simulink model "meat_1024pt_bee2"  (Simulink 6.2)
settings: Solver=ode45  StartTime=0.0  StopTime=60000  RelTol=1e-3
undefined symbols (not defined in the file): BEE2_usr, bit_rev, pfb_coeff_gen_calc
libraries: xbsIndex_r3 x1083, casper_library x93, xps_library x28
(part 1 of 8)
settings Model: LastModifiedBy=siemion
settings DebuggingCC: SolverPrmCheckMsg=warning

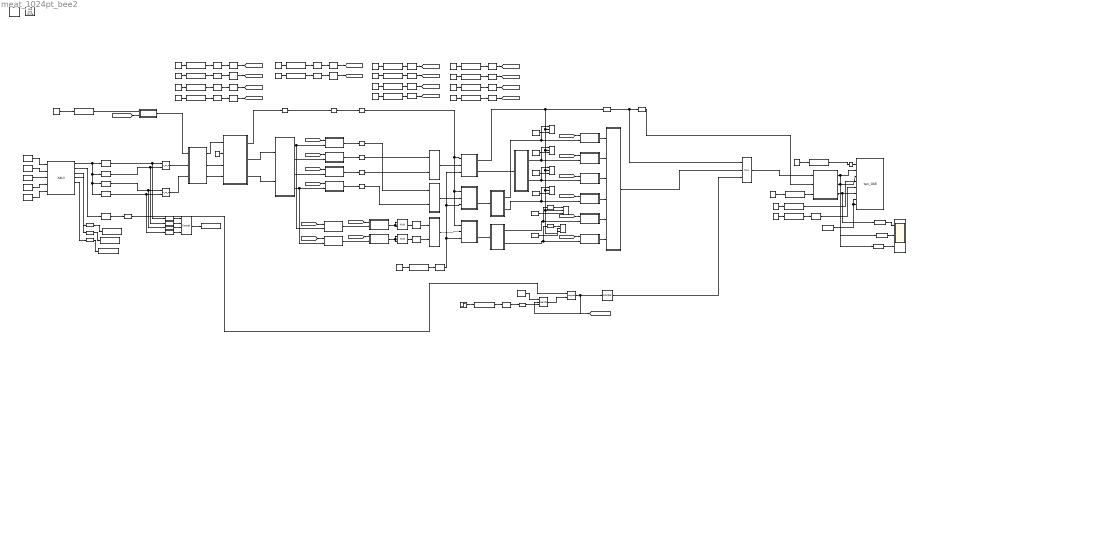
== system meat_1024pt_bee2 ==
  note: left
  note: ATA Kurtosis Machine
      | Author: Andrew Siemion
      | Author: Peter McMahon
      | Version: 1.0
      | August 2009
  note: n * LCM(taps*clksperFFT=4*1024=2048,
      | clksperacc=(acclen+1)*veclen=5*2048=10240)=20480
  note: XAUI Output:
      |
      | outofband[0]: 100PPS
      | outofband[1]: 1PPS
      |
      | data[0-7]: Pol 1 I
      | data[8-15]: Pol 1 Q
      | data[16-23]: Pol 2 I
      | data[24-31]: Pol 2 Q
      | data[31-63]: unused
  note: min acclen for serializer = # of parallel inputs
  note: XAUI Scope
      | Outputs raw bits from XAUI so you can measure voltage levels
  note: ARM/PPS Reset Circuit
      | 1. User sets ARM high at half-second
      | 2. 1PPS arrives.
      | 3. PPSARMReset signal goes high for one clock on the 1PPS
      | 4. ARM is reset, and won't go high again until user brings it low then high
  note: Unsigned, 18-bits, b.p. at 12
      | Coefficient by which to scale the output of the Stokes Detector.
  note: Extract 8 bits from 32
      | (latency: 1)
      | Don't delay valid since we will prepend a counter
      | and extend valid for one clock
  note: When "valid" goes high, it's the start of a
      | packet, so insert a counter.
      |
      | Note that since the bitselect_i subsystems each have a delay of 1,
      | valid goes high 1 clock before the data arrives.
  note: Need valid to be high while data is valid (1024 clocks), and
      | one extra clock for the "header" (counter). Total clocks: 1025.
  note: end-of-frame goes high for the last clock
      | that valid is high. This is a requirement for
      | the 10GbE block to work.
  note: ** Sending out data every second clock.
      | 10GbE tx_data input is 64 bits wide.
      | We only produce 32-bits of data per clock.
      | Therefore we must buffer 32-bits every second clock
      | and concat it with the current data output to get 64-bits
      | every second clock. The tx_valid line is modified to
      | accommodate this.
  note: Intended usage:
      | Connect to 108MHz bandwidth beamformer.
      | Input: I,Q 108MSa/sec, dual polarization.
      |   i.e. 8-bits I, 8-bits Q, x2 pol = 32 bits
      | Runs synchronously (i.e. assumes 32-bits
      | arrives from XAUI every FPGA clock)
  note: Selects which 8-bits from 32 are outputted.
      | 0 is lowest 8-bits.
      | 3 is highest 8-bits.
  note: Powers are unsigned and cross-terms are signed.
      | Hence we have to use separate accumulators for
      | them.
  note: Unsigned, 18-bits, b.p. at 12
      | Coefficient by which to scale the output of the Stokes Detector.
  note: Packet Size is in bytes / eight
  " System Generator" : xbsIndex_r3/ System Generator  Tag=genX  xilinxfamily=Virtex2P  part=xc2vp50  speed=-7  package=ff1152  synthesis_tool=XST  directory=./meat_1024pt_lwip_reg/sysgen  testbench=off  simulink_period=1  sysclk_period=8  incr_netlist=off  trim_vbits=Everywhere in SubSystem  dbl_ovrd=According to Block Masks  core_generation=According to Block Masks  run_coregen=off  deprecated_control=off  eval_field=0
      settings: AttributesFormatString=System\nGenerator
  Constant : Constant  Value=4000
  Constant1 : Constant  Value=4000
  Constant{10,15..17} (4 alike) : Constant  Value=0
  Constant{3..6,11..12} (6 alike) : Constant  Value=2^12
  Constant2 : Constant  Value=2
  Constant7 : Constant
  Constant8 : Constant
  Constant9 : Constant
  Convert : xbsIndex_r3/Convert  arith_type=Unsigned  n_bits=32  bin_pt=0  quantization=Truncate  overflow=Wrap  latency=0  explicit_period=on  period=1  dbl_ovrd=off  show_param=off  inserted_by_tool=off  pipeline=off
      settings: xl_area=[0, 0, 0, 0, 0, 0, 0]
  Convert1 : xbsIndex_r3/Convert  arith_type=Unsigned  n_bits=32  bin_pt=0  quantization=Truncate  overflow=Wrap  latency=0  explicit_period=on  period=1  dbl_ovrd=off  show_param=off  inserted_by_tool=off  pipeline=off
      settings: xl_area=[0, 0, 0, 0, 0, 0, 0]
  Convert2 : xbsIndex_r3/Convert  arith_type=Unsigned  n_bits=32  bin_pt=0  quantization=Truncate  overflow=Wrap  latency=0  explicit_period=on  period=1  dbl_ovrd=off  show_param=off  inserted_by_tool=off  pipeline=off
      settings: xl_area=[0, 0, 0, 0, 0, 0, 0]
  Gateway Out1 : xbsIndex_r3/Gateway Out  output_type=Double  nbits=8  bin_pt=6  arith_type=Boolean  quantization=Truncate  overflow=Wrap  hdl_port=on  timing_constraint=None  locs_specified=off  LOCs={}  needs_fixed_name=off  show_param=off
      settings: xl_area=[0, 0, 0, 0, 0, 0, 0]
  Gateway Out2 : xbsIndex_r3/Gateway Out  output_type=Double  nbits=8  bin_pt=6  arith_type=Boolean  quantization=Truncate  overflow=Wrap  hdl_port=on  timing_constraint=None  locs_specified=off  LOCs={}  needs_fixed_name=off  show_param=off
      settings: xl_area=[0, 0, 0, 0, 0, 0, 0]
  Gateway Out3 : xbsIndex_r3/Gateway Out  output_type=Double  nbits=8  bin_pt=6  arith_type=Boolean  quantization=Truncate  overflow=Wrap  hdl_port=on  timing_constraint=None  locs_specified=off  LOCs={}  needs_fixed_name=off  show_param=off
      settings: xl_area=[0, 0, 0, 0, 0, 0, 0]
  Packet_Size : xps_library/software register  Tag=xps:sw_reg  io_dir=From Processor  arith_type=Unsigned  bitwidth=32  bin_pt=0  sample_period=1  gw_name=meat_1024pt_bee2_Packet_Size_user_data_out
  Packetizer : Subsystem
  Scope : Scope  NumInputPorts=3
      settings: YMin=0~0~0  YMax=1~1~9500
  Slice : xbsIndex_r3/Slice  mode=Lower Bit Location + Width  nbits=20  bit1=0  base1=MSB of Input  bit0=0  base0=LSB of Input  boolean_output=off  explicit_period=off  period=1  dbl_ovrd=off
  Slice1 : xbsIndex_r3/Slice  mode=Lower Bit Location + Width  nbits=16  bit1=0  base1=MSB of Input  bit0=0  base0=LSB of Input  boolean_output=off  explicit_period=off  period=1  dbl_ovrd=off
  Slice{10,15..17} (4 alike) : xbsIndex_r3/Slice  mode=Lower Bit Location + Width  nbits=3  bit1=0  base1=MSB of Input  bit0=0  base0=LSB of Input  boolean_output=off  explicit_period=off  period=1  dbl_ovrd=off
  Slice{3..4,7..8,11..12} (6 alike) : xbsIndex_r3/Slice  mode=Lower Bit Location + Width  nbits=18  bit1=0  base1=MSB of Input  bit0=0  base0=LSB of Input  boolean_output=off  explicit_period=off  period=1  dbl_ovrd=off
  Slice{2,5..6,9} (4 alike) : xbsIndex_r3/Slice  mode=Lower Bit Location + Width  nbits=2  bit1=0  base1=MSB of Input  bit0=0  base0=LSB of Input  boolean_output=off  explicit_period=off  period=1  dbl_ovrd=off
  StokesDetector : Subsystem
  XAUI : xps_library/XAUI  Tag=xps:xaui  demux=1  port=BEE2_usr:0  show_param=on  pre_emph=2  swing=800
  XSG core config : xps_library/XSG core config  Tag=xps:xsg  hw_sys=BEE2_usr  ibob_linux=off  clk_src=usr_clk2x  gpio_clk_io_group=iBOB:sma  gpio_clk_bit_index=0  clk_rate=125  sample_period=1  synthesis_tool=XST  mpc_type=powerpc405
  bitselect_1 : Subsystem
  bitselect_5 : Subsystem
  cns0_{,1..5} (6 alike) : xbsIndex_r3/Constant  const=0  equ=P=C  arith_type=Boolean  n_bits=1  bin_pt=0  opselect=C  inp2=PCIN>>17  opr=+  inp1=P  carry=CIN  iostate=0  explicit_period=on  period=1  dbl_ovrd=off
  cns_10GbE : xbsIndex_r3/Constant  const=0  equ=P=C  arith_type=Boolean  n_bits=32  bin_pt=0  opselect=C  inp2=PCIN>>17  opr=+  inp1=P  carry=CIN  iostate=0  explicit_period=on  period=1  dbl_ovrd=off
  cns_acclen : Constant  Value=4
  cns_reset : xbsIndex_r3/Constant  const=1  equ=P=C  arith_type=Boolean  n_bits=1  bin_pt=0  opselect=C  inp2=PCIN>>17  opr=+  inp1=P  carry=CIN  iostate=0  explicit_period=on  period=1  dbl_ovrd=off
  cns_sync_period : Constant  Value=10240
  cns_sync_period1 : Constant  Value=205
  cns_sync_period2 : Constant  Value=0
  cns_xaui_rx_get : xbsIndex_r3/Constant  const=1  equ=P=C  arith_type=Boolean  n_bits=1  bin_pt=0  opselect=C  inp2=PCIN>>17  opr=+  inp1=P  carry=CIN  iostate=0  explicit_period=on  period=1  dbl_ovrd=off
  cns_xaui_rx_reset : xbsIndex_r3/Constant  const=0  equ=P=C  arith_type=Boolean  n_bits=1  bin_pt=0  opselect=C  inp2=PCIN>>17  opr=+  inp1=P  carry=CIN  iostate=0  explicit_period=on  period=1  dbl_ovrd=off
  cns_xaui_tx_data : xbsIndex_r3/Constant  const=0  equ=P=C  arith_type=Unsigned  n_bits=64  bin_pt=0  opselect=C  inp2=PCIN>>17  opr=+  inp1=P  carry=CIN  iostate=0  explicit_period=on  period=1  dbl_ovrd=off
  cns_xaui_tx_outofband : xbsIndex_r3/Constant  const=0  equ=P=C  arith_type=Unsigned  n_bits=8  bin_pt=0  opselect=C  inp2=PCIN>>17  opr=+  inp1=P  carry=CIN  iostate=0  explicit_period=on  period=1  dbl_ovrd=off
  cns_xaui_tx_valid : xbsIndex_r3/Constant  const=0  equ=P=C  arith_type=Boolean  n_bits=8  bin_pt=0  opselect=C  inp2=PCIN>>17  opr=+  inp1=P  carry=CIN  iostate=0  explicit_period=on  period=1  dbl_ovrd=off
  coeff_delay : xbsIndex_r3/Delay  latency=6  reg_retiming=off  explicit_period=off  period=1  en=off  accept_only_valid=off  init_zero=on  dbl_ovrd=off  show_param=off
      settings: xl_area=[0, 0, 0, 0, 0, 0, 0]
  concat_xauiscope : xbsIndex_r3/Concat  num_inputs=4  explicit_period=off  period=1  dbl_ovrd=off
  cram1 : Subsystem  AncestorBlock=gavrt_library/cram  mask(cram){num_slice=6}
      mask prompts: num_slice "Number of slices"
      mask help: Concatenates inputs together after forcing binary point to zero.
      mask init:
      | cram_init(gcb, ...
      |     'num_slice', num_slice);
  cram_crossterms : Subsystem  AncestorBlock=gavrt_library/cram  mask(cram){num_slice=2}
      mask prompts: num_slice "Number of slices"
      mask help: Concatenates inputs together after forcing binary point to zero.
      mask init:
      | cram_init(gcb, ...
      |     'num_slice', num_slice);
  cram_kurt : Subsystem  AncestorBlock=gavrt_library/cram  mask(cram){num_slice=2}
      mask prompts: num_slice "Number of slices"
      mask help: Concatenates inputs together after forcing binary point to zero.
      mask init:
      | cram_init(gcb, ...
      |     'num_slice', num_slice);
  cram_powers : Subsystem  AncestorBlock=gavrt_library/cram  mask(cram){num_slice=2}
      mask prompts: num_slice "Number of slices"
      mask help: Concatenates inputs together after forcing binary point to zero.
      mask init:
      | cram_init(gcb, ...
      |     'num_slice', num_slice);
  fft : Subsystem  AncestorBlock=casper_library/FFTs/fft  mask(fft){FFTSize=10, BitWidth=18, n_inputs=0, quantization=Truncate, overflow=Wrap, add_latency=3, mult_latency=4, bram_latency=3}
      mask prompts: FFTSize "Size of FFT: (2^?)"; BitWidth "Bit Width"; n_inputs "Number of Simultaneous Inputs: (2^?)"; quantization "Quantization Behavior"; overflow "Overflow Behavior"; add_latency "Add Latency"; mult_latency "Mult Latency"; bram_latency "BRAM Latency"
      mask init:
      | fft_init(gcb,...
      |     'FFTSize', FFTSize,...
      |     'BitWidth', BitWidth,...
      |     'n_inputs', n_inputs,...
      |     'quantization', quantization,...
      |     'overflow', overflow,...
      |     'add_latency', add_latency,...
      |     'mult_latency', mult_latency,...
      |     'bram_latency', bram_latency);
      settings: AttributesFormatString=FFTSize=10, n_inputs=0
      mask StyleString: edit,edit,edit,popup(Truncate|Round  (unbiased: +/- Inf)|Round  (unbiased: Even Values)),popup(Wrap|Saturate|Error),edit,edit,edit
  force_adc_i{0..3} (4 alike) : xbsIndex_r3/Reinterpret  force_arith_type=on  arith_type=Unsigned  force_bin_pt=on  bin_pt=0  force_valid=on
  kurt_delay{1..5} (5 alike) : xbsIndex_r3/Delay  latency=5  reg_retiming=on  explicit_period=off  period=1  en=off  accept_only_valid=off  init_zero=on  dbl_ovrd=off  show_param=off
      settings: xl_area=[0, 0, 0, 0, 0, 0, 0]
  kurt_output1a : xps_library/software register  Tag=xps:sw_reg  io_dir=From Processor  arith_type=Unsigned  bitwidth=32  bin_pt=0  sample_period=1  gw_name=meat_1024pt_bee2_kurt_output1a_user_data_out
  kurt_output1b : xps_library/software register  Tag=xps:sw_reg  io_dir=From Processor  arith_type=Unsigned  bitwidth=32  bin_pt=0  sample_period=1  gw_name=meat_1024pt_bee2_kurt_output1b_user_data_out
  kurt_scale_1a : xps_library/software register  Tag=xps:sw_reg  io_dir=From Processor  arith_type=Unsigned  bitwidth=32  bin_pt=0  sample_period=1  gw_name=meat_1024pt_bee2_kurt_scale_1a_user_data_out
  kurt_scale_1b : xps_library/software register  Tag=xps:sw_reg  io_dir=From Processor  arith_type=Unsigned  bitwidth=32  bin_pt=0  sample_period=1  gw_name=meat_1024pt_bee2_kurt_scale_1b_user_data_out
  kurt_select1a : xps_library/software register  Tag=xps:sw_reg  io_dir=From Processor  arith_type=Unsigned  bitwidth=32  bin_pt=0  sample_period=1  gw_name=meat_1024pt_bee2_kurt_select1a_user_data_out
  kurt_select1b : xps_library/software register  Tag=xps:sw_reg  io_dir=From Processor  arith_type=Unsigned  bitwidth=32  bin_pt=0  sample_period=1  gw_name=meat_1024pt_bee2_kurt_select1b_user_data_out
  log_arm_pps : xbsIndex_r3/Logical  logical_function=AND  inputs=2  precision=Full  arith_type=Unsigned  n_bits=8  bin_pt=2  align_bp=on  latency=0  explicit_period=off  period=1  en=off  dbl_ovrd=off  show_param=off
      settings: xl_area=[0, 0, 0, 0, 0, 0, 0]
  mux_counter_data : xbsIndex_r3/Mux  inputs=2  precision=Full  arith_type="Signed  (2's comp)"  n_bits=8  bin_pt=2  quantization=Truncate  overflow=Wrap  latency=1  explicit_period=off  period=1  en=off  dbl_ovrd=off  show_param=off  mux_type=off  use_rpm=off  gen_core=off
      settings: xl_area=[0, 0, 0, 0, 0, 0, 0]
  pfb_fir : Subsystem  AncestorBlock=casper_library/PFBs/pfb_fir  mask(pfb_fir){PFBSize=10, TotalTaps=4, WindowType=hamming, n_inputs=0, MakeBiplex=1, BitWidthIn=8, BitWidthOut=18, CoeffBitWidth=8, CoeffDistMem=1, add_latency=2, mult_latency=3, bram_latency=3, quantization=Truncate, fwidth=1}
      mask prompts: PFBSize "Size of PFB: (2^? pnts)"; TotalTaps "Total Number of Taps:"; WindowType "Windowing Function:"; n_inputs "Number of Simultaneous Inputs: (2^?)"; MakeBiplex "Make Biplex"; BitWidthIn "Input Bitwidth:"; BitWidthOut "Output Bitwidth:"; CoeffBitWidth "Coefficient Bitwidth:"; CoeffDistMem "Use Distributed Memory for Coeffs"; add_latency "Add Latency"; mult_latency "Mult Latency"; bram_latency "BRAM Latency"; quantization "Quantization Behavior"; fwidth "Bin Width Scaling (normal=1)"
      mask init:
      | pfb_fir_init(gcb, ...
      |     'PFBSize', PFBSize, ...
      |     'TotalTaps', TotalTaps, ...
      |     'WindowType', WindowType, ...
      |     'n_inputs', n_inputs, ...
      |     'MakeBiplex', MakeBiplex, ...
      |     'BitWidthIn', BitWidthIn, ...
      |     'BitWidthOut', BitWidthOut, ...
      |     'CoeffBitWidth', CoeffBitWidth, ...
      |     'CoeffDistMem', CoeffDistMem, ...
      |     'add_latency', add_latency, ...
      |     'mult_latency', mult_latency, ...
      |     'bram_latency', bram_latency, ...
      |     'quantization', quantization, ...
      |     'fwidth', fwidth);
      settings: AttributesFormatString=taps=4, add_latency=2
      mask StyleString: edit,edit,popup(bartlett|barthannwin|blackman|blackmanharris|bohamwin|chebwin|flattopwin|gausswin|hamming|hann|kaiser|nuttallwin|parzenwin|rectwin|tukeywin|triang),edit,edit,edit,edit,edit,edit,edit,edit,edit,popup(Truncate|Round  (unbiased: +/- Inf)|Round  (unbiased: Even Values)),edit
  pol1_kurt1 : Subsystem
  pol2_kurt1 : Subsystem
  posedge : casper_library/Misc/posedge  Tag=Rising Edge Detector
  posedge_arm : casper_library/Misc/posedge  Tag=Rising Edge Detector
  posedge_pps_xaui : casper_library/Misc/posedge  Tag=Rising Edge Detector
  power1_1 : xbsIndex_r3/Mult  precision=User Defined  arith_type=Unsigned  n_bits=32  bin_pt=0  quantization="Round  (unbiased: +/- Inf)"  overflow=Saturate  latency=4  explicit_period=off  period=1  en=off  dbl_ovrd=off  show_param=on  mult_type=Parallel  oversample=1  use_embedded=off  pipeline=on  use_rpm=on  placement_style=Rectangular Shape  gen_core=off
      settings: xl_area=[0, 0, 0, 0, 0, 0, 0]
  power1_2 : xbsIndex_r3/Mult  precision=User Defined  arith_type=Unsigned  n_bits=32  bin_pt=0  quantization="Round  (unbiased: +/- Inf)"  overflow=Saturate  latency=4  explicit_period=off  period=1  en=off  dbl_ovrd=off  show_param=on  mult_type=Parallel  oversample=1  use_embedded=off  pipeline=on  use_rpm=on  placement_style=Rectangular Shape  gen_core=off
      settings: xl_area=[0, 0, 0, 0, 0, 0, 0]
  pulse_ext_valid_output : casper_library/Misc/pulse_ext  pulse_len=1025
  reg_10GbE_destport0 : xps_library/software register  Tag=xps:sw_reg  io_dir=From Processor  arith_type=Unsigned  bitwidth=32  bin_pt=0  sample_period=1  gw_name=meat_1024pt_bee2_reg_10GbE_destport0_user_data_out
  reg_acclen : xps_library/software register  Tag=xps:sw_reg  io_dir=From Processor  arith_type=Unsigned  bitwidth=32  bin_pt=0  sample_period=1  gw_name=meat_1024pt_bee2_reg_acclen_user_data_out
  reg_arm : xps_library/software register  Tag=xps:sw_reg  io_dir=From Processor  arith_type=Unsigned  bitwidth=32  bin_pt=0  sample_period=1  gw_name=meat_1024pt_bee2_reg_arm_user_data_out
  reg_coeff_stokes1 : xps_library/software register  Tag=xps:sw_reg  io_dir=From Processor  arith_type=Unsigned  bitwidth=32  bin_pt=0  sample_period=1  gw_name=meat_1024pt_bee2_reg_coeff_stokes1_user_data_out
  reg_coeff_stokes2 : xps_library/software register  Tag=xps:sw_reg  io_dir=From Processor  arith_type=Unsigned  bitwidth=32  bin_pt=0  sample_period=1  gw_name=meat_1024pt_bee2_reg_coeff_stokes2_user_data_out
  reg_coeff_stokes3 : xps_library/software register  Tag=xps:sw_reg  io_dir=From Processor  arith_type=Unsigned  bitwidth=32  bin_pt=0  sample_period=1  gw_name=meat_1024pt_bee2_reg_coeff_stokes3_user_data_out
  reg_coeff_stokes4 : xps_library/software register  Tag=xps:sw_reg  io_dir=From Processor  arith_type=Unsigned  bitwidth=32  bin_pt=0  sample_period=1  gw_name=meat_1024pt_bee2_reg_coeff_stokes4_user_data_out
  reg_ip : xps_library/software register  Tag=xps:sw_reg  io_dir=From Processor  arith_type=Unsigned  bitwidth=32  bin_pt=0  sample_period=1  gw_name=meat_1024pt_bee2_reg_ip_user_data_out
  reg_output_bitselect1 : xps_library/software register  Tag=xps:sw_reg  io_dir=From Processor  arith_type=Unsigned  bitwidth=32  bin_pt=0  sample_period=1  gw_name=meat_1024pt_bee2_reg_output_bitselect1_user_data_out
  reg_output_bitselect2 : xps_library/software register  Tag=xps:sw_reg  io_dir=From Processor  arith_type=Unsigned  bitwidth=32  bin_pt=0  sample_period=1  gw_name=meat_1024pt_bee2_reg_output_bitselect2_user_data_out
  reg_output_bitselect3 : xps_library/software register  Tag=xps:sw_reg  io_dir=From Processor  arith_type=Unsigned  bitwidth=32  bin_pt=0  sample_period=1  gw_name=meat_1024pt_bee2_reg_output_bitselect3_user_data_out
  reg_output_bitselect4 : xps_library/software register  Tag=xps:sw_reg  io_dir=From Processor  arith_type=Unsigned  bitwidth=32  bin_pt=0  sample_period=1  gw_name=meat_1024pt_bee2_reg_output_bitselect4_user_data_out
  reg_reset_arm : xbsIndex_r3/Register  init=0  reg_only_valid=off  explicit_period=on  period=1  rst=on  en=on  out_en=off  dbl_ovrd=off  show_param=off
      settings: xl_area=[0, 0, 0, 0, 0, 0, 0]
  reg_sync_period : xps_library/software register  Tag=xps:sw_reg  io_dir=From Processor  arith_type=Unsigned  bitwidth=32  bin_pt=0  sample_period=1  gw_name=meat_1024pt_bee2_reg_sync_period_user_data_out
  reg_xauiscope : xps_library/software register  Tag=xps:sw_reg  io_dir=To Processor  arith_type=Unsigned  bitwidth=32  bin_pt=0  sample_period=1  gw_name=meat_1024pt_bee2_reg_xauiscope_user_data_in
  reint{,1..5} (6 alike) : xbsIndex_r3/Reinterpret  force_arith_type=on  arith_type=Unsigned  force_bin_pt=on  bin_pt=12  force_valid=on
  reint_bp_0 : xbsIndex_r3/Reinterpret  force_arith_type=on  arith_type=Unsigned  force_bin_pt=on  bin_pt=23  force_valid=on
  reint_bp_1 : xbsIndex_r3/Reinterpret  force_arith_type=on  arith_type=Unsigned  force_bin_pt=on  bin_pt=23  force_valid=on
  ri_to_c : casper_library/Misc/ri_to_c
  ri_to_c1 : casper_library/Misc/ri_to_c
  rx_empty : xps_library/software register  Tag=xps:sw_reg  io_dir=To Processor  arith_type=Unsigned  bitwidth=32  bin_pt=0  sample_period=1  gw_name=meat_1024pt_bee2_rx_empty_user_data_in
  rx_linkdown : xps_library/software register  Tag=xps:sw_reg  io_dir=To Processor  arith_type=Unsigned  bitwidth=32  bin_pt=0  sample_period=1  gw_name=meat_1024pt_bee2_rx_linkdown_user_data_in
  rx_valid : xps_library/software register  Tag=xps:sw_reg  io_dir=To Processor  arith_type=Unsigned  bitwidth=32  bin_pt=0  sample_period=1  gw_name=meat_1024pt_bee2_rx_valid_user_data_in
  shift : xbsIndex_r3/Constant  const=-1  equ=P=C  arith_type="Signed  (2's comp)"  n_bits=32  bin_pt=0  opselect=C  inp2=PCIN>>17  opr=+  inp1=P  carry=CIN  iostate=0  explicit_period=on  period=1  dbl_ovrd=off
  signed_bitselect_2 : Subsystem
  signed_bitselect_3 : Subsystem
  signed_scale2 : Subsystem
  signed_scale3 : Subsystem
  sim_step_arm : Step  SampleTime=0
  slc_arm : xbsIndex_r3/Slice  mode=Lower Bit Location + Width  nbits=1  bit1=0  base1=MSB of Input  bit0=0  base0=LSB of Input  boolean_output=on  explicit_period=off  period=1  dbl_ovrd=off
  slc_bitselect_1 : xbsIndex_r3/Slice  mode=Upper Bit Location + Width  nbits=32  bit1=0  base1=MSB of Input  bit0=0  base0=MSB of Input  boolean_output=off  explicit_period=off  period=1  dbl_ovrd=off
  slc_bitselect_2 : xbsIndex_r3/Slice  mode=Upper Bit Location + Width  nbits=32  bit1=0  base1=MSB of Input  bit0=0  base0=MSB of Input  boolean_output=off  explicit_period=off  period=1  dbl_ovrd=off
  slc_bitselect_3 : xbsIndex_r3/Slice  mode=Lower Bit Location + Width  nbits=1  bit1=0  base1=LSB of Input  bit0=0  base0=LSB of Input  boolean_output=on  explicit_period=off  period=1  dbl_ovrd=off
  slc_xaui_data_pol1_I : xbsIndex_r3/Slice  mode=Lower Bit Location + Width  nbits=8  bit1=0  base1=MSB of Input  bit0=0  base0=LSB of Input  boolean_output=off  explicit_period=off  period=1  dbl_ovrd=off
  slc_xaui_data_pol1_Q : xbsIndex_r3/Slice  mode=Lower Bit Location + Width  nbits=8  bit1=0  base1=MSB of Input  bit0=8  base0=LSB of Input  boolean_output=off  explicit_period=off  period=1  dbl_ovrd=off
  slc_xaui_data_pol2_I : xbsIndex_r3/Slice  mode=Lower Bit Location + Width  nbits=8  bit1=0  base1=MSB of Input  bit0=16  base0=LSB of Input  boolean_output=off  explicit_period=off  period=1  dbl_ovrd=off
  slc_xaui_data_pol2_Q : xbsIndex_r3/Slice  mode=Lower Bit Location + Width  nbits=8  bit1=0  base1=MSB of Input  bit0=24  base0=LSB of Input  boolean_output=off  explicit_period=off  period=1  dbl_ovrd=off
  slc_xaui_outofband_1pps : xbsIndex_r3/Slice  mode=Lower Bit Location + Width  nbits=1  bit1=0  base1=MSB of Input  bit0=1  base0=LSB of Input  boolean_output=on  explicit_period=off  period=1  dbl_ovrd=off
  snap_vacc_{1..6} (6 alike) : casper_library/Scopes/snap  nsamples=11
  stokes_delay : xbsIndex_r3/Delay  latency=5  reg_retiming=off  explicit_period=off  period=1  en=off  accept_only_valid=off  init_zero=on  dbl_ovrd=off  show_param=off
      settings: xl_area=[0, 0, 0, 0, 0, 0, 0]
  sync_generator : Subsystem
  system_counter : xbsIndex_r3/Counter  cnt_type=Free Running  n_bits=64  bin_pt=0  arith_type=Unsigned  start_count=0  cnt_to=Inf  cnt_by_val=1  operation=Up  explicit_period=off  period=1  load_pin=off  rst=on  en=off  dbl_ovrd=off  show_param=off  use_rpm=on  gen_core=off
      settings: xl_area=[0, 0, 0, 0, 0, 0, 0]
  tGbE_reset : xps_library/software register  Tag=xps:sw_reg  io_dir=From Processor  arith_type=Unsigned  bitwidth=32  bin_pt=0  sample_period=1  gw_name=meat_1024pt_bee2_tGbE_reset_user_data_out
  ten_GbE0 : xps_library/ten_GbE  Tag=xps:tengbe  port=BEE2_usr:3  mac_lite=off  show_param=on  pre_emph=2  swing=800
  uncram_crossterms : Subsystem  AncestorBlock=gavrt_library/uncram  mask(uncram){num_slice=2, slice_width=32, bin_pt=23, arith_type=1}
      mask prompts: num_slice "Number of slices"; slice_width "Slice Width"; bin_pt "Output Binary Point"; arith_type "Output Arithmetic Type (0=Unsigned, 1=Signed, 2=Boolean)"
      mask help: Takes a concatenated input and slices it up into even pieces and reinterprets them as signed fixed point numbers with a given binary point.
      mask init:
      | uncram_init(gcb, ...
      |     'num_slice', num_slice, ...
      |     'slice_width', slice_width, ...
      |     'bin_pt', bin_pt, ...
      |     'arith_type', arith_type);
      settings: AttributesFormatString=Fix_32_23
  uncram_powers : Subsystem  AncestorBlock=gavrt_library/uncram  mask(uncram){num_slice=2, slice_width=32, bin_pt=23, arith_type=0}
      mask prompts: num_slice "Number of slices"; slice_width "Slice Width"; bin_pt "Output Binary Point"; arith_type "Output Arithmetic Type (0=Unsigned, 1=Signed, 2=Boolean)"
      mask help: Takes a concatenated input and slices it up into even pieces and reinterprets them as signed fixed point numbers with a given binary point.
      mask init:
      | uncram_init(gcb, ...
      |     'num_slice', num_slice, ...
      |     'slice_width', slice_width, ...
      |     'bin_pt', bin_pt, ...
      |     'arith_type', arith_type);
      settings: AttributesFormatString=UFix_32_23
  uncram_powers1 : Subsystem  AncestorBlock=gavrt_library/uncram  mask(uncram){num_slice=2, slice_width=48, bin_pt=23, arith_type=0}
      mask prompts: num_slice "Number of slices"; slice_width "Slice Width"; bin_pt "Output Binary Point"; arith_type "Output Arithmetic Type (0=Unsigned, 1=Signed, 2=Boolean)"
      mask help: Takes a concatenated input and slices it up into even pieces and reinterprets them as signed fixed point numbers with a given binary point.
      mask init:
      | uncram_init(gcb, ...
      |     'num_slice', num_slice, ...
      |     'slice_width', slice_width, ...
      |     'bin_pt', bin_pt, ...
      |     'arith_type', arith_type);
      settings: AttributesFormatString=UFix_48_23
  unsigned_bitselect_1 : Subsystem
  unsigned_bitselect_2 : Subsystem
  unsigned_bitselect_3 : Subsystem
  unsigned_bitselect_4 : Subsystem
  unsigned_scale1 : Subsystem
  unsigned_scale2 : Subsystem
  vacc : Subsystem  AncestorBlock=gavrt_library/vacc  mask(vacc){veclen=10, ninputs=2, max_accum=8, arith_type=1, in_bit_width=24, in_bin_pt=23, out_bit_width=32, out_bin_pt=23, register_din=1, add_latency=2, bram_latency=2, mux_latency=1}
      mask prompts: veclen "Vector Length (2^?)"; ninputs "Number of Simultaneous Vectors"; max_accum "Maximum # Accumulations (2^?)"; arith_type "Arithmetic Type (0=Unsigned, 1=Signed)"; in_bit_width "Input Bit Width"; in_bin_pt "Input Binary Point"; out_bit_width "Output Bit Width"; out_bin_pt "Output Binary Point"; register_din "Register Input Data  (1 = Enable Register Retiming on input delay)"; add_latency "Add Latency"; bram_latency "BRAM Latency"; mux_latency "Mux Latency"
      mask help:
      | Sync is expected the clock before the first data to be accumulated.
      | Use the Cram block to feed din for multiple simultaneous inputs.
      | acc_len is the number of vectors to sum.
      | valid is high while a valid accumulation is being clocked out on dout.
      | If only one sync pulse is provided, valid accumulations will repeatedly appear on dout as they become available.
      | Undesired behavior may occur if acc_len is changed without a new sync pulse.
      | Note: The output is an unsigned concatenation of the output streams. Thus, even with only one stream, the output must be recast before using.
      | Register Input Data controls the "Enable Register Retiming" parameter of the delays on 'din'.
      mask init:
      | vacc_init(gcb, ...
      |     'veclen', veclen, ...
      |     'ninputs', ninputs, ...
      |     'max_accum', max_accum, ...
      |     'arith_type', arith_type, ...
      |     'in_bit_width', in_bit_width, ...
      |     'in_bin_pt', in_bin_pt, ...
      |     'out_bit_width', out_bit_width, ...
      |     'out_bin_pt', out_bin_pt, ...
      |     'register_din', register_din, ...
      |     'add_latency', add_latency, ...
      |     'bram_latency', bram_latency, ...
      |     'mux_latency', mux_latency);
      settings: AttributesFormatString=|
      | vector length=1024, inputs=2
      | max accumulations=2^8
  vacc1 : Subsystem  AncestorBlock=gavrt_library/vacc  mask(vacc){veclen=10, ninputs=2, max_accum=8, arith_type=0, in_bit_width=24, in_bin_pt=23, out_bit_width=32, out_bin_pt=23, register_din=1, add_latency=2, bram_latency=2, mux_latency=1}
      mask prompts: veclen "Vector Length (2^?)"; ninputs "Number of Simultaneous Vectors"; max_accum "Maximum # Accumulations (2^?)"; arith_type "Arithmetic Type (0=Unsigned, 1=Signed)"; in_bit_width "Input Bit Width"; in_bin_pt "Input Binary Point"; out_bit_width "Output Bit Width"; out_bin_pt "Output Binary Point"; register_din "Register Input Data  (1 = Enable Register Retiming on input delay)"; add_latency "Add Latency"; bram_latency "BRAM Latency"; mux_latency "Mux Latency"
      mask help:
      | Sync is expected the clock before the first data to be accumulated.
      | Use the Cram block to feed din for multiple simultaneous inputs.
      | acc_len is the number of vectors to sum.
      | valid is high while a valid accumulation is being clocked out on dout.
      | If only one sync pulse is provided, valid accumulations will repeatedly appear on dout as they become available.
      | Undesired behavior may occur if acc_len is changed without a new sync pulse.
      | Note: The output is an unsigned concatenation of the output streams. Thus, even with only one stream, the output must be recast before using.
      | Register Input Data controls the "Enable Register Retiming" parameter of the delays on 'din'.
      mask init: same as meat_1024pt_bee2/vacc
      settings: AttributesFormatString=|
      | vector length=1024, inputs=2
      | max accumulations=2^8
  vacc2 : Subsystem  AncestorBlock=gavrt_library/vacc  mask(vacc){veclen=10, ninputs=2, max_accum=8, arith_type=0, in_bit_width=32, in_bin_pt=23, out_bit_width=48, out_bin_pt=23, register_din=1, add_latency=2, bram_latency=2, mux_latency=1}
      mask prompts: veclen "Vector Length (2^?)"; ninputs "Number of Simultaneous Vectors"; max_accum "Maximum # Accumulations (2^?)"; arith_type "Arithmetic Type (0=Unsigned, 1=Signed)"; in_bit_width "Input Bit Width"; in_bin_pt "Input Binary Point"; out_bit_width "Output Bit Width"; out_bin_pt "Output Binary Point"; register_din "Register Input Data  (1 = Enable Register Retiming on input delay)"; add_latency "Add Latency"; bram_latency "BRAM Latency"; mux_latency "Mux Latency"
      mask help:
      | Sync is expected the clock before the first data to be accumulated.
      | Use the Cram block to feed din for multiple simultaneous inputs.
      | acc_len is the number of vectors to sum.
      | valid is high while a valid accumulation is being clocked out on dout.
      | If only one sync pulse is provided, valid accumulations will repeatedly appear on dout as they become available.
      | Undesired behavior may occur if acc_len is changed without a new sync pulse.
      | Note: The output is an unsigned concatenation of the output streams. Thus, even with only one stream, the output must be recast before using.
      | Register Input Data controls the "Enable Register Retiming" parameter of the delays on 'din'.
      mask init: same as meat_1024pt_bee2/vacc
      settings: AttributesFormatString=|
      | vector length=1024, inputs=2
      | max accumulations=2^8
  wires:
  Slice/1 -> vacc/3(acc_len), vacc1/3(acc_len), vacc2/3(acc_len)
  stokes_delay/1 -> coeff_delay/1
  reg_sync_period/1 -> sync_generator/1(period)
  sync_generator/1(sync) -> pfb_fir/1(sync)
  reg_acclen/1 -> Slice/1
  cns_acclen/1 -> reg_acclen/1
  cns_sync_period/1 -> reg_sync_period/1
  reg_10GbE_destport0/1 -> Slice1/1
  Constant/1 -> reg_10GbE_destport0/1
  Slice1/1 -> ten_GbE0/5
  Constant1/1 -> reg_ip/1
  reg_ip/1 -> ten_GbE0/4
  [PPSARMReset] -> sync_generator/2(reset)
  reg_arm/1 -> slc_arm/1
  cns_reset/1 -> reg_reset_arm/1
  reg_reset_arm/1 -> log_arm_pps/2
  log_arm_pps/1 -> reg_reset_arm/2, system_counter/1, [PPSARMReset]
  slc_arm/1 -> posedge_arm/1
  posedge_arm/1 -> reg_reset_arm/3
  concat_xauiscope/1 -> reg_xauiscope/1
  force_adc_i0/1 -> concat_xauiscope/1
  force_adc_i1/1 -> concat_xauiscope/2
  force_adc_i2/1 -> concat_xauiscope/3
  force_adc_i3/1 -> concat_xauiscope/4
  sim_step_arm/1 -> reg_arm/1
  Constant3/1 -> reg_coeff_stokes1/1
  reg_coeff_stokes1/1 -> Slice3/1
  Slice3/1 -> reint/1
  signed_bitselect_2/1(data_out) -> cram1/2(In2)
  signed_bitselect_3/1(data_out) -> cram1/3(In3)
  unsigned_bitselect_4/1(data_out) -> cram1/4(In4)
  vacc/1(valid) -> posedge/1, snap_vacc_1/2, snap_vacc_2/2, snap_vacc_3/2, snap_vacc_4/2, snap_vacc_5/2, snap_vacc_6/2
  system_counter/1 -> mux_counter_data/3
  posedge/1 -> pulse_ext_valid_output/1, mux_counter_data/1
  pulse_ext_valid_output/1 -> Packetizer/2(Data Start)
  ri_to_c/1 -> pfb_fir/2(pol1_in1)
  ri_to_c1/1 -> pfb_fir/3(pol2_in1)
  pfb_fir/1(sync_out) -> fft/1(sync)
  shift/1 -> fft/2(shift)
  pfb_fir/2(pol1_out1) -> fft/3(pol0)
  pfb_fir/3(pol2_out1) -> fft/4(pol1)
  fft/1(sync_out) -> stokes_delay/1
  fft/2(out0) -> StokesDetector/1(pol1_f0)
  fft/3(out1) -> StokesDetector/2(pol2_f0)
  coeff_delay/1 -> kurt_delay1/1
  StokesDetector/1(f0_pol1_pow) -> unsigned_scale1/2(data_in), pol1_kurt1/2(data_in)
  StokesDetector/2(f0_x_re) -> signed_scale2/2(data_in)
  StokesDetector/3(f0_x_im) -> signed_scale3/2(data_in)
  StokesDetector/4(f0_pol2_pow) -> unsigned_scale2/2(data_in), pol2_kurt1/2(data_in)
  reint/1 -> [StokesCoeff1]
  Constant4/1 -> reg_coeff_stokes2/1
  reg_coeff_stokes2/1 -> Slice4/1
  Slice4/1 -> reint1/1
  reint1/1 -> [StokesCoeff2]
  Constant5/1 -> reg_coeff_stokes3/1
  reg_coeff_stokes3/1 -> Slice7/1
  Slice7/1 -> reint2/1
  reint2/1 -> [StokesCoeff3]
  Constant6/1 -> reg_coeff_stokes4/1
  reg_coeff_stokes4/1 -> Slice8/1
  Slice8/1 -> reint3/1
  reint3/1 -> [StokesCoeff4]
  [StokesCoeff1] -> unsigned_scale1/1(coeff)
  [StokesCoeff2] -> signed_scale2/1(coeff)
  [StokesCoeff3] -> signed_scale3/1(coeff)
  [StokesCoeff4] -> unsigned_scale2/1(coeff)
  Constant2/1 -> reg_output_bitselect1/1
  reg_output_bitselect1/1 -> Slice2/1
  signed_scale2/1(data_out) -> kurt_delay3/1
  signed_scale3/1(data_out) -> kurt_delay4/1
  cram_crossterms/1(Out) -> vacc/2(din)
  cram_powers/1(Out) -> vacc1/2(din)
  unsigned_scale1/1(data_out) -> kurt_delay2/1
  unsigned_scale2/1(data_out) -> kurt_delay5/1
  uncram_crossterms/1(Out1) -> signed_bitselect_2/2(data_in), snap_vacc_2/1
  uncram_crossterms/2(Out2) -> signed_bitselect_3/2(data_in), snap_vacc_3/1
  vacc/2(dout) -> uncram_crossterms/1(In)
  vacc1/2(dout) -> uncram_powers/1(In)
  uncram_powers/1(Out1) -> unsigned_bitselect_1/2(data_in), snap_vacc_1/1
  unsigned_bitselect_1/1(data_out) -> cram1/1(In1)
  Constant7/1 -> reg_output_bitselect2/1
  reg_output_bitselect2/1 -> Slice5/1
  Constant8/1 -> reg_output_bitselect3/1
  reg_output_bitselect3/1 -> Slice6/1
  Constant9/1 -> reg_output_bitselect4/1
  reg_output_bitselect4/1 -> Slice9/1
  Slice2/1 -> [BitSelect1]
  Slice5/1 -> [BitSelect2]
  Slice6/1 -> [BitSelect3]
  Slice9/1 -> [BitSelect4]
  [BitSelect1] -> unsigned_bitselect_1/1(bitselect)
  uncram_powers/2(Out2) -> unsigned_bitselect_4/2(data_in), snap_vacc_4/1
  [BitSelect4] -> unsigned_bitselect_4/1(bitselect)
  [BitSelect3] -> signed_bitselect_3/1(bitselect)
  [BitSelect2] -> signed_bitselect_2/1(bitselect)
  XAUI/1 -> slc_xaui_data_pol1_I/1, slc_xaui_data_pol1_Q/1, slc_xaui_data_pol2_I/1, slc_xaui_data_pol2_Q/1
  slc_xaui_data_pol1_I/1 -> ri_to_c/1, force_adc_i0/1
  slc_xaui_data_pol1_Q/1 -> ri_to_c/2, force_adc_i1/1
  slc_xaui_data_pol2_I/1 -> ri_to_c1/1, force_adc_i2/1
  slc_xaui_data_pol2_Q/1 -> ri_to_c1/2, force_adc_i3/1
  cns_xaui_rx_get/1 -> XAUI/1
  cns_xaui_rx_reset/1 -> XAUI/2
  cns_xaui_tx_data/1 -> XAUI/3
  cns_xaui_tx_outofband/1 -> XAUI/4
  cns_xaui_tx_valid/1 -> XAUI/5
  slc_xaui_outofband_1pps/1 -> posedge_pps_xaui/1
  XAUI/2 -> slc_xaui_outofband_1pps/1
  cns0_/1 -> snap_vacc_1/3
  cns0_1/1 -> snap_vacc_2/3
  cns0_2/1 -> snap_vacc_3/3
  cns0_3/1 -> snap_vacc_4/3
  Constant10/1 -> kurt_select1a/1
  kurt_select1a/1 -> Slice10/1
  bitselect_5/1(data_out) -> power1_2/1, power1_2/2
  bitselect_1/1(data_out) -> power1_1/1, power1_1/2
  power1_2/1 -> reint_bp_0/1
  power1_1/1 -> reint_bp_1/1
  Constant11/1 -> kurt_scale_1a/1
  kurt_scale_1a/1 -> Slice11/1
  Slice11/1 -> reint4/1
  reint4/1 -> [kurtscale1a]
  Constant12/1 -> kurt_scale_1b/1
  kurt_scale_1b/1 -> Slice12/1
  Slice12/1 -> reint5/1
  reint5/1 -> [kurtscale1b]
  Slice10/1 -> [kurtbitselect1a]
  [kurtbitselect1a] -> bitselect_5/1(bitselect)
  [kurtbitselect1b] -> bitselect_1/1(bitselect)
  pol2_kurt1/1(data_out) -> bitselect_1/2(data_in)
  pol1_kurt1/1(data_out) -> bitselect_5/2(data_in)
  Constant15/1 -> kurt_select1b/1
  kurt_select1b/1 -> Slice15/1
  Slice15/1 -> [kurtbitselect1b]
  [kurtscale1b] -> pol2_kurt1/1(coeff)
  [kurtscale1a] -> pol1_kurt1/1(coeff)
  kurt_delay2/1 -> cram_powers/1(In1)
  kurt_delay3/1 -> cram_crossterms/1(In1)
  kurt_delay4/1 -> cram_crossterms/2(In2)
  kurt_delay5/1 -> cram_powers/2(In2)
  cram_kurt/1(Out) -> vacc2/2(din)
  reint_bp_0/1 -> cram_kurt/1(In1)
  reint_bp_1/1 -> cram_kurt/2(In2)
  vacc2/2(dout) -> uncram_powers1/1(In)
  unsigned_bitselect_2/1(data_out) -> cram1/5(In5)
  [kurtoutput1a] -> unsigned_bitselect_2/1(bitselect)
  unsigned_bitselect_3/1(data_out) -> cram1/6(In6)
  [kurtoutput1b] -> unsigned_bitselect_3/1(bitselect)
  Constant16/1 -> kurt_output1a/1
  kurt_output1a/1 -> Slice16/1
  Slice16/1 -> [kurtoutput1a]
  Constant17/1 -> kurt_output1b/1
  kurt_output1b/1 -> Slice17/1
  Slice17/1 -> [kurtoutput1b]
  uncram_powers1/1(Out1) -> unsigned_bitselect_2/2(data_in), slc_bitselect_1/1
  uncram_powers1/2(Out2) -> unsigned_bitselect_3/2(data_in), slc_bitselect_2/1
  cns0_4/1 -> snap_vacc_5/3
  cns0_5/1 -> snap_vacc_6/3
  cram1/1(Out) -> mux_counter_data/2
  Packet_Size/1 -> Packetizer/3(Packet Size)
  cns_sync_period1/1 -> Packet_Size/1
  Packetizer/3(End of Frame) -> ten_GbE0/6, Gateway Out3/1
  Packetizer/2(Data Valid) -> ten_GbE0/3, Gateway Out2/1
  Packetizer/1(Data Out) -> ten_GbE0/2, Gateway Out1/1
  mux_counter_data/1 -> Packetizer/1(Data In)
  kurt_delay1/1 -> vacc/1(sync), vacc1/1(sync), vacc2/1(sync)
  slc_bitselect_2/1 -> snap_vacc_6/1
  slc_bitselect_1/1 -> snap_vacc_5/1
  Convert/1 -> rx_empty/1
  Convert1/1 -> rx_valid/1
  Convert2/1 -> rx_linkdown/1
  XAUI/5 -> Convert2/1
  XAUI/4 -> Convert1/1
  XAUI/3 -> Convert/1
  Gateway Out3/1 -> Scope/1
  Gateway Out2/1 -> Scope/2
  Gateway Out1/1 -> Scope/3
  cns_10GbE/1 -> ten_GbE0/7, ten_GbE0/8
  cns_sync_period2/1 -> tGbE_reset/1
  tGbE_reset/1 -> slc_bitselect_3/1
  slc_bitselect_3/1 -> ten_GbE0/1
  posedge_pps_xaui/1 -> log_arm_pps/1

== system meat_1024pt_bee2/Packetizer ==
  Data In : Inport  Port=1  LatchInput=off
  Data Start : Inport  Port=2  LatchInput=off
  Packet Size : Inport  Port=3  LatchInput=off
  Convert : xbsIndex_r3/Convert  arith_type=Boolean  n_bits=8  bin_pt=6  quantization=Truncate  overflow=Wrap  latency=1  explicit_period=off  period=1  dbl_ovrd=off  show_param=off  inserted_by_tool=off  pipeline=off
      settings: xl_area=[0, 0, 0, 0, 0, 0, 0]
  Counter1 : xbsIndex_r3/Counter  cnt_type=Free Running  n_bits=32  bin_pt=0  arith_type=Unsigned  start_count=1  cnt_to=Inf  cnt_by_val=1  operation=Up  explicit_period=on  period=1  load_pin=off  rst=on  en=on  dbl_ovrd=off  show_param=off  use_rpm=on  gen_core=off
      settings: xl_area=[0, 0, 0, 0, 0, 0, 0]
  Delay : xbsIndex_r3/Delay  latency=1  reg_retiming=off  explicit_period=off  period=1  en=off  accept_only_valid=off  init_zero=on  dbl_ovrd=off  show_param=off
      settings: xl_area=[0, 0, 0, 0, 0, 0, 0]
  Delay1 : xbsIndex_r3/Delay  latency=2  reg_retiming=off  explicit_period=off  period=1  en=off  accept_only_valid=off  init_zero=on  dbl_ovrd=off  show_param=off
      settings: xl_area=[0, 0, 0, 0, 0, 0, 0]
  Delay2 : xbsIndex_r3/Delay  latency=2  reg_retiming=off  explicit_period=off  period=1  en=off  accept_only_valid=off  init_zero=on  dbl_ovrd=off  show_param=off
      settings: xl_area=[0, 0, 0, 0, 0, 0, 0]
  Logical : xbsIndex_r3/Logical  logical_function=OR  inputs=2  precision=Full  arith_type=Unsigned  n_bits=8  bin_pt=2  align_bp=on  latency=0  explicit_period=off  period=1  en=off  dbl_ovrd=off  show_param=off
      settings: xl_area=[0, 0, 0, 0, 0, 0, 0]
  Relational2 : xbsIndex_r3/Relational  mode=a>=b  latency=1  explicit_period=off  period=1  en=off  dbl_ovrd=off  show_param=off
      settings: xl_area=[0, 0, 0, 0, 0, 0, 0]
  cns1 : xbsIndex_r3/Constant  const=4  equ=P=C  arith_type=Unsigned  n_bits=3  bin_pt=0  opselect=C  inp2=PCIN>>17  opr=+  inp1=P  carry=CIN  iostate=0  explicit_period=off  period=1  dbl_ovrd=off
  period_sub : xbsIndex_r3/AddSub  mode=Subtraction  precision=User Defined  arith_type=Unsigned  n_bits=32  bin_pt=0  quantization=Truncate  overflow=Wrap  latency=0  explicit_period=off  period=1  use_carryin=off  use_carryout=off  en=off  dbl_ovrd=off  show_param=off  use_core=on  pipeline=off  use_rpm=on  gen_core=off
      settings: xl_area=[0, 0, 0, 0, 0, 0, 0]
  posedge : casper_library/Misc/posedge  Tag=Rising Edge Detector
  posedge1 : casper_library/Misc/posedge  Tag=Rising Edge Detector
  pulse_ext_valid_output : casper_library/Misc/pulse_ext  pulse_len=1025
  Data Out : Outport
  Data Valid : Outport  Port=2
  End of Frame : Outport  Port=3
  wires:
  Delay/1 -> pulse_ext_valid_output/1
  Delay1/1 -> Counter1/2
  Logical/1 -> Counter1/1
  pulse_ext_valid_output/1 -> Delay1/1, Data Valid/1
  posedge1/1 -> Logical/1, Delay/1
  period_sub/1 -> Relational2/2
  Convert/1 -> posedge/1, Logical/2
  Relational2/1 -> Convert/1
  Counter1/1 -> Relational2/1
  cns1/1 -> period_sub/2
  Data In/1 -> Delay2/1
  Delay2/1 -> Data Out/1
  posedge/1 -> End of Frame/1
  Data Start/1 -> posedge1/1
  Packet Size/1 -> period_sub/1

== system meat_1024pt_bee2/StokesDetector ==
  pol1_f0 : Inport  Port=1  LatchInput=off
  pol2_f0 : Inport  Port=2  LatchInput=off
  XMultiply_f0 : Subsystem
  pol1_power0 : Subsystem
  pol2_power0 : Subsystem
  f0_pol1_pow : Outport
  f0_x_re : Outport  Port=2
  f0_x_im : Outport  Port=3
  f0_pol2_pow : Outport  Port=4
  wires:
  pol1_f0/1 -> XMultiply_f0/1(Pol1), pol1_power0/1(c)
  pol2_f0/1 -> XMultiply_f0/2(Pol2), pol2_power0/1(c)
  pol1_power0/1(power) -> f0_pol1_pow/1
  XMultiply_f0/1(X Real) -> f0_x_re/1
  XMultiply_f0/2(X Imag) -> f0_x_im/1
  pol2_power0/1(power) -> f0_pol2_pow/1

== system meat_1024pt_bee2/bitselect_1 ==
  bitselect : Inport  Port=1  LatchInput=off
  data_in : Inport  Port=2  LatchInput=off
  mux_bitselect : xbsIndex_r3/Mux  inputs=6  precision=Full  arith_type="Signed  (2's comp)"  n_bits=8  bin_pt=2  quantization=Truncate  overflow=Wrap  latency=1  explicit_period=off  period=1  en=off  dbl_ovrd=off  show_param=off  mux_type=off  use_rpm=off  gen_core=off
      settings: xl_area=[0, 0, 0, 0, 0, 0, 0]
  reint_bp_0 : xbsIndex_r3/Reinterpret  force_arith_type=on  arith_type=Unsigned  force_bin_pt=on  bin_pt=0  force_valid=on
  slc_bitselect_1 : xbsIndex_r3/Slice  mode=Lower Bit Location + Width  nbits=18  bit1=0  base1=MSB of Input  bit0=0  base0=LSB of Input  boolean_output=off  explicit_period=off  period=1  dbl_ovrd=off
  slc_bitselect_2 : xbsIndex_r3/Slice  mode=Lower Bit Location + Width  nbits=18  bit1=0  base1=MSB of Input  bit0=1  base0=LSB of Input  boolean_output=off  explicit_period=off  period=1  dbl_ovrd=off
  slc_bitselect_3 : xbsIndex_r3/Slice  mode=Lower Bit Location + Width  nbits=18  bit1=0  base1=MSB of Input  bit0=2  base0=LSB of Input  boolean_output=off  explicit_period=off  period=1  dbl_ovrd=off
  slc_bitselect_4 : xbsIndex_r3/Slice  mode=Lower Bit Location + Width  nbits=18  bit1=0  base1=MSB of Input  bit0=3  base0=LSB of Input  boolean_output=off  explicit_period=off  period=1  dbl_ovrd=off
  slc_bitselect_5 : xbsIndex_r3/Slice  mode=Lower Bit Location + Width  nbits=18  bit1=0  base1=MSB of Input  bit0=4  base0=LSB of Input  boolean_output=off  explicit_period=off  period=1  dbl_ovrd=off
  slc_bitselect_6 : xbsIndex_r3/Slice  mode=Lower Bit Location + Width  nbits=18  bit1=0  base1=MSB of Input  bit0=5  base0=LSB of Input  boolean_output=off  explicit_period=off  period=1  dbl_ovrd=off
  data_out : Outport
  wires:
  slc_bitselect_6/1 -> mux_bitselect/7
  slc_bitselect_5/1 -> mux_bitselect/6
  slc_bitselect_4/1 -> mux_bitselect/5
  reint_bp_0/1 -> slc_bitselect_1/1, slc_bitselect_6/1, slc_bitselect_5/1, slc_bitselect_4/1, slc_bitselect_3/1, slc_bitselect_2/1
  mux_bitselect/1 -> data_out/1
  bitselect/1 -> mux_bitselect/1
  data_in/1 -> reint_bp_0/1
  slc_bitselect_3/1 -> mux_bitselect/4
  slc_bitselect_2/1 -> mux_bitselect/3
  slc_bitselect_1/1 -> mux_bitselect/2

== system meat_1024pt_bee2/bitselect_5 ==
  bitselect : Inport  Port=1  LatchInput=off
  data_in : Inport  Port=2  LatchInput=off
  mux_bitselect : xbsIndex_r3/Mux  inputs=6  precision=Full  arith_type="Signed  (2's comp)"  n_bits=8  bin_pt=2  quantization=Truncate  overflow=Wrap  latency=1  explicit_period=off  period=1  en=off  dbl_ovrd=off  show_param=off  mux_type=off  use_rpm=off  gen_core=off
      settings: xl_area=[0, 0, 0, 0, 0, 0, 0]
  reint_bp_0 : xbsIndex_r3/Reinterpret  force_arith_type=on  arith_type=Unsigned  force_bin_pt=on  bin_pt=0  force_valid=on
  slc_bitselect_1 : xbsIndex_r3/Slice  mode=Lower Bit Location + Width  nbits=18  bit1=0  base1=MSB of Input  bit0=0  base0=LSB of Input  boolean_output=off  explicit_period=off  period=1  dbl_ovrd=off
  slc_bitselect_2 : xbsIndex_r3/Slice  mode=Lower Bit Location + Width  nbits=18  bit1=0  base1=MSB of Input  bit0=1  base0=LSB of Input  boolean_output=off  explicit_period=off  period=1  dbl_ovrd=off
  slc_bitselect_3 : xbsIndex_r3/Slice  mode=Lower Bit Location + Width  nbits=18  bit1=0  base1=MSB of Input  bit0=2  base0=LSB of Input  boolean_output=off  explicit_period=off  period=1  dbl_ovrd=off
  slc_bitselect_4 : xbsIndex_r3/Slice  mode=Lower Bit Location + Width  nbits=18  bit1=0  base1=MSB of Input  bit0=3  base0=LSB of Input  boolean_output=off  explicit_period=off  period=1  dbl_ovrd=off
  slc_bitselect_5 : xbsIndex_r3/Slice  mode=Lower Bit Location + Width  nbits=18  bit1=0  base1=MSB of Input  bit0=4  base0=LSB of Input  boolean_output=off  explicit_period=off  period=1  dbl_ovrd=off
  slc_bitselect_6 : xbsIndex_r3/Slice  mode=Lower Bit Location + Width  nbits=18  bit1=0  base1=MSB of Input  bit0=5  base0=LSB of Input  boolean_output=off  explicit_period=off  period=1  dbl_ovrd=off
  data_out : Outport
  wires:
  slc_bitselect_1/1 -> mux_bitselect/2
  slc_bitselect_2/1 -> mux_bitselect/3
  slc_bitselect_3/1 -> mux_bitselect/4
  data_in/1 -> reint_bp_0/1
  bitselect/1 -> mux_bitselect/1
  mux_bitselect/1 -> data_out/1
  reint_bp_0/1 -> slc_bitselect_2/1, slc_bitselect_3/1, slc_bitselect_4/1, slc_bitselect_5/1, slc_bitselect_6/1, slc_bitselect_1/1
  slc_bitselect_4/1 -> mux_bitselect/5
  slc_bitselect_5/1 -> mux_bitselect/6
  slc_bitselect_6/1 -> mux_bitselect/7

== system meat_1024pt_bee2/cram1 ==
  In1 : Inport  Port=1  LatchInput=off
  In2 : Inport  Port=2  LatchInput=off
  In3 : Inport  Port=3  LatchInput=off
  In4 : Inport  Port=4  LatchInput=off
  In5 : Inport  Port=5  LatchInput=off
  In6 : Inport  Port=6  LatchInput=off
  Concat : S-Function  AncestorBlock=xbsIndex_r3/Concat  FunctionName=xlconcat  Parameters=sfcn_mwsv__  mask(Xilinx Bus Concatenator){num_inputs=6, explicit_period=off, period=1, dbl_ovrd=off}
      mask prompts: num_inputs "Number of Inputs"; explicit_period "Use Explicit Sample Period"; period "Sample Period  (use -1 to inherit first known input period)"; dbl_ovrd "Override with Doubles"
      mask help: Concatenates two or more inputs. Inputs must be unsigned with binary point at zero.
      mask init:
      | [designRoot, family, part, speed, package, simulinkPeriod, sysclkPeriod, dbl_ovrd, trimVbit] = xlSysgenSettings(gcb,1,1);
      | [bg,fg] = xlcmap('XBlock',dbl_ovrd);
      | iPos = get_param(gcb,'Position');
      | iWidth=iPos(3)-iPos(1); iHeight=iPos(4)-iPos(2);
      | iCx=iWidth/2;
      | iCy=iHeight/2;
      | [logoX, logoY] = xlogo(iPos);
      | 
      | 
      | 
      | 
      | % one time added for param list
      | numInputs = num_inputs + 1;
      | precision0 = 1;
      | latency = 0;
      | dblOvrd = dbl_ovrd;
      | explicitClk = explicit_period;
      | 
      | 
      | % just pass everything to s-function
      | sfcn_mwsv__ = get_param(gcb, 'MaskWSVariables');
      mask Help: eval('xlWeb(xlhtmldoclink(''Concat''))');
      mask StyleString: popup(2|3|4|5|6|7|8|9|10|11|12|13|14|15|16),checkbox,edit,checkbox
      mask CallbackString: |xlMagicCallback||
      mask Display:
      | patch([0 iWidth iWidth 0],[0 0 iHeight iHeight] , bg);
      | patch(logoX,logoY, fg);
      | port_label('input',1,'hi');
      | port_label('input',num_inputs+1,'lo');
      | port_label('output',1,'cat');
      | ;plot([0 0 iWidth iWidth 0], [0 iHeight iHeight 0 0]);
  Reinterp{1..6} (6 alike) : xbsIndex_r3/Reinterpret  force_arith_type=on  arith_type=Unsigned  force_bin_pt=on  bin_pt=0  force_valid=on
  Out : Outport
  wires:
  Concat/1 -> Out/1
  In1/1 -> Reinterp1/1
  Reinterp1/1 -> Concat/1
  In2/1 -> Reinterp2/1
  Reinterp2/1 -> Concat/2
  In3/1 -> Reinterp3/1
  Reinterp3/1 -> Concat/3
  In4/1 -> Reinterp4/1
  Reinterp4/1 -> Concat/4
  In5/1 -> Reinterp5/1
  Reinterp5/1 -> Concat/5
  In6/1 -> Reinterp6/1
  Reinterp6/1 -> Concat/6
